simulink subsystem "guidance_law_subsystem"  (R2021b)
settings: Solver=VariableStepAuto  StartTime=0.0  StopTime=10.0  RelTol=1e-3
values from neighbouring files (symbols this model uses):
  d2r = pi/180    (= 0.0174532925199)    [PN_Guidance_matlab.m]
libraries: simulink x1
settings Model: Creator=rocke  LastModifiedBy=rocke

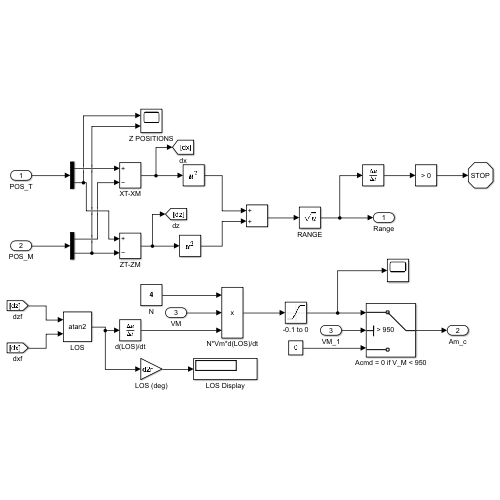
[thumbnail: Simulink's stored preview of the top-level diagram]
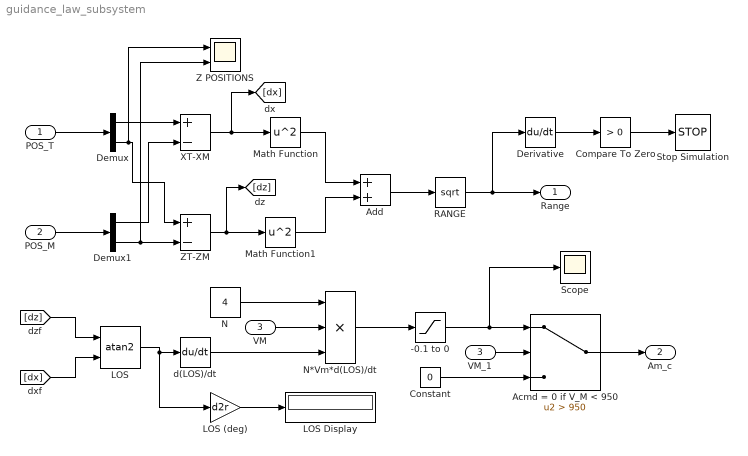
== system guidance_law_subsystem ==
  POS_T : Inport
  POS_M : Inport  Port=2
  VM : Inport  Port=3
  -0.1 to 0 : Saturate  UpperLimit=0  LowerLimit=-0.05
  Acmd = 0 if V_M < 950 : Switch  Criteria=u2 > Threshold  Threshold=950
  Add : Sum
  Compare To Zero : simulink/Logic and Bit Operations/Compare To Zero  relop=>  OutDataTypeStr=boolean
  Constant : Constant  Value=0
  Demux : Demux  Outputs=2
  Demux1 : Demux  Outputs=2
  Derivative : Derivative
  LOS : Trigonometry  Operator=atan2
  LOS (deg) : Gain  Gain=d2r
  LOS Display : Display
  Math Function : Math  Operator=square  SaturateOnIntegerOverflow=on
  Math Function1 : Math  Operator=square  SaturateOnIntegerOverflow=on
  N : Constant  Value=4
  N*Vm*d(LOS)/dt : Product  Inputs=3
  RANGE : Sqrt  SaturateOnIntegerOverflow=on
  Scope : Scope
  Stop Simulation : Stop
  VM_1 : InportShadow  Port=3
  XT-XM : Sum  Inputs=+-
  Z POSITIONS : Scope  NumInputPorts=2
  ZT-ZM : Sum  Inputs=+-
  d(LOS)/dt : Derivative
  Range : Outport
  Am_c : Outport  Port=2
  wires:
  Acmd = 0 if V_M < 950/1 -> Am_c/1
  VM_1/1 -> Acmd = 0 if V_M < 950/2
  POS_M/1 -> Demux1/1
  Demux/1 -> XT-XM/1
  N/1 -> N*Vm*d(LOS)/dt/1
  VM/1 -> N*Vm*d(LOS)/dt/2
  Derivative/1 -> Compare To Zero/1
  [dx] -> LOS/2
  N*Vm*d(LOS)/dt/1 -> -0.1 to 0/1
  Demux1/1 -> XT-XM/2
  Add/1 -> RANGE/1
  Constant/1 -> Acmd = 0 if V_M < 950/3
  Demux/2 -> Z POSITIONS/1, ZT-ZM/1
  RANGE/1 -> Range/1, Derivative/1
  XT-XM/1 -> [dx], Math Function/1
  [dz] -> LOS/1
  Compare To Zero/1 -> Stop Simulation/1
  LOS (deg)/1 -> LOS Display/1
  Math Function1/1 -> Add/2
  POS_T/1 -> Demux/1
  -0.1 to 0/1 -> Scope/1, Acmd = 0 if V_M < 950/1
  Math Function/1 -> Add/1
  ZT-ZM/1 -> [dz], Math Function1/1
  Demux1/2 -> Z POSITIONS/2, ZT-ZM/2
  LOS/1 -> LOS (deg)/1, d(LOS)/dt/1
  d(LOS)/dt/1 -> N*Vm*d(LOS)/dt/3
